simulink model "skarab_adc4x3g_14"  (R2018a)
settings: Solver=VariableStepAuto  StartTime=0.0  StopTime=10.0  RelTol=1e-3
libraries: xbsIndex_r4 x76
settings Model: Creator=qwerty40  LastModifiedBy=clifford
settings CodeAppCC: StateflowObjectComments=on

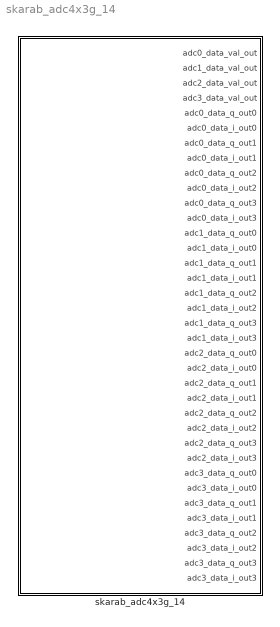
== system skarab_adc4x3g_14 ==
  skarab_adc4x3g_14 : Subsystem  Tag=xps:skarab_adc4x3g_14  mask(hmc){mez=2, sync_ms=Master}
      mask prompts: mez "Mezzanine slot"; sync_ms "Master/Slave"
      mask help: Interface to ADC cards available on SKARAB boards.
      mask init:
      | skarab_adc4x3g_14_mask(gcb);
      mask TypeOptions mez: 0 | 1 | 2 | 3
      mask TypeOptions sync_ms: Master | Slave
      mask DialogControl Container6 Prompt: Parameters

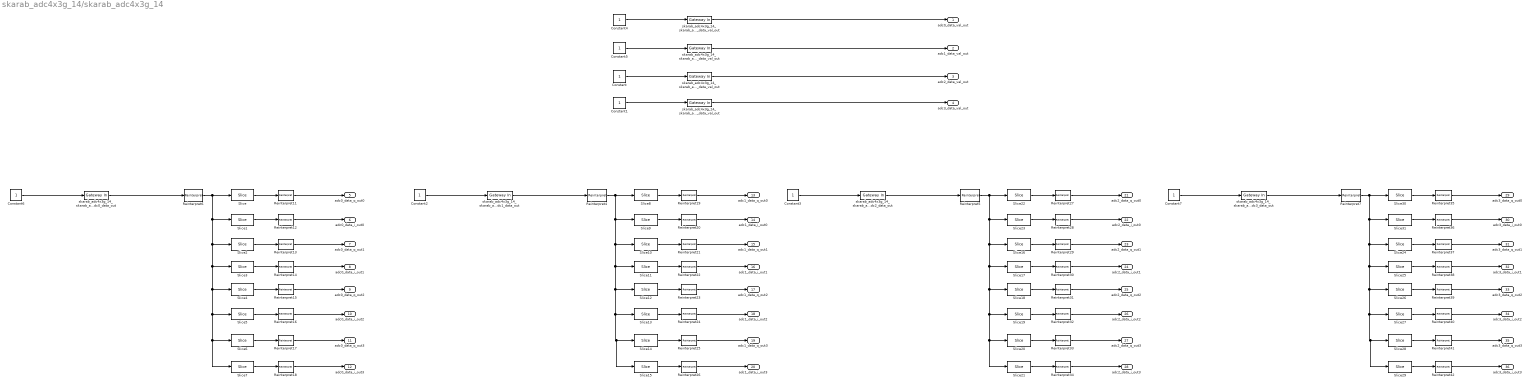
== system skarab_adc4x3g_14/skarab_adc4x3g_14 ==
  Constant{,1..7} (8 alike) : Constant
  Reinterpret{11..42} (32 alike) : xbsIndex_r4/Reinterpret  force_arith_type=on  arith_type="Signed  (2's comp)"  force_bin_pt=on  bin_pt=15  block_type=reinterpret
  Reinterpret{4..7} (4 alike) : xbsIndex_r4/Reinterpret  force_arith_type=on  arith_type=Unsigned  force_bin_pt=on  bin_pt=0  block_type=reinterpret
  Slice{,8,22,30} (4 alike) : xbsIndex_r4/Slice  nbits=16  boolean_output=off  mode=Lower Bit Location + Width  bit1=0  base1=MSB of Input  bit0=0  base0=LSB of Input  dbl_ovrd=off  block_type=slice
  Slice{1,9,23,31} (4 alike) : xbsIndex_r4/Slice  nbits=16  boolean_output=off  mode=Lower Bit Location + Width  bit1=0  base1=MSB of Input  bit0=16  base0=LSB of Input  dbl_ovrd=off  block_type=slice
  Slice{2,10,16,24} (4 alike) : xbsIndex_r4/Slice  nbits=16  boolean_output=off  mode=Lower Bit Location + Width  bit1=0  base1=MSB of Input  bit0=32  base0=LSB of Input  dbl_ovrd=off  block_type=slice
  Slice{3,11,17,25} (4 alike) : xbsIndex_r4/Slice  nbits=16  boolean_output=off  mode=Lower Bit Location + Width  bit1=0  base1=MSB of Input  bit0=48  base0=LSB of Input  dbl_ovrd=off  block_type=slice
  Slice{4,12,18,26} (4 alike) : xbsIndex_r4/Slice  nbits=16  boolean_output=off  mode=Lower Bit Location + Width  bit1=0  base1=MSB of Input  bit0=64  base0=LSB of Input  dbl_ovrd=off  block_type=slice
  Slice{5,13,19,27} (4 alike) : xbsIndex_r4/Slice  nbits=16  boolean_output=off  mode=Lower Bit Location + Width  bit1=0  base1=MSB of Input  bit0=80  base0=LSB of Input  dbl_ovrd=off  block_type=slice
  Slice{6,14,20,28} (4 alike) : xbsIndex_r4/Slice  nbits=16  boolean_output=off  mode=Lower Bit Location + Width  bit1=0  base1=MSB of Input  bit0=96  base0=LSB of Input  dbl_ovrd=off  block_type=slice
  Slice{7,15,21,29} (4 alike) : xbsIndex_r4/Slice  nbits=16  boolean_output=off  mode=Lower Bit Location + Width  bit1=0  base1=MSB of Input  bit0=112  base0=LSB of Input  dbl_ovrd=off  block_type=slice
  skarab_adc4x3g_14_skarab_adc4x3g_14_adc0_data_out : xbsIndex_r4/Gateway In  gui_display_data_type=Fixed-point  arith_type=Unsigned  n_bits=128  bin_pt=0  preci_type=Single  exp_width=8  frac_width=24  rows=1  columns=1  quantization=Truncate  overflow=Wrap  period=1  UseAsADC=off  ADCChannel='1'  interface=None  automatic_assignment=on  address_offset=hex2dec('00')  intf_name=''  intf_description=''  default_value=0  timing_constraint=None  locs_specified=off  LOCs={}  io_standard={}  inherit_from_input=off  hdl_port=on  dbl_ovrd=off  block_type=gatewayin
  skarab_adc4x3g_14_skarab_adc4x3g_14_adc0_data_val_out : xbsIndex_r4/Gateway In  gui_display_data_type=Boolean  arith_type=Boolean  n_bits=16  bin_pt=14  preci_type=Single  exp_width=8  frac_width=24  rows=1  columns=1  quantization="Round  (unbiased: +/- Inf)"  overflow=Saturate  period=1  UseAsADC=off  ADCChannel='1'  interface=None  automatic_assignment=on  address_offset=hex2dec('00')  intf_name=''  intf_description=''  default_value=0  timing_constraint=None  locs_specified=off  LOCs={}  io_standard={}  inherit_from_input=off  hdl_port=on  dbl_ovrd=off  block_type=gatewayin
  skarab_adc4x3g_14_skarab_adc4x3g_14_adc1_data_out : xbsIndex_r4/Gateway In  gui_display_data_type=Fixed-point  arith_type=Unsigned  n_bits=128  bin_pt=0  preci_type=Single  exp_width=8  frac_width=24  rows=1  columns=1  quantization=Truncate  overflow=Wrap  period=1  UseAsADC=off  ADCChannel='1'  interface=None  automatic_assignment=on  address_offset=hex2dec('00')  intf_name=''  intf_description=''  default_value=0  timing_constraint=None  locs_specified=off  LOCs={}  io_standard={}  inherit_from_input=off  hdl_port=on  dbl_ovrd=off  block_type=gatewayin
  skarab_adc4x3g_14_skarab_adc4x3g_14_adc1_data_val_out : xbsIndex_r4/Gateway In  gui_display_data_type=Boolean  arith_type=Boolean  n_bits=16  bin_pt=14  preci_type=Single  exp_width=8  frac_width=24  rows=1  columns=1  quantization="Round  (unbiased: +/- Inf)"  overflow=Saturate  period=1  UseAsADC=off  ADCChannel='1'  interface=None  automatic_assignment=on  address_offset=hex2dec('00')  intf_name=''  intf_description=''  default_value=0  timing_constraint=None  locs_specified=off  LOCs={}  io_standard={}  inherit_from_input=off  hdl_port=on  dbl_ovrd=off  block_type=gatewayin
  skarab_adc4x3g_14_skarab_adc4x3g_14_adc2_data_out : xbsIndex_r4/Gateway In  gui_display_data_type=Fixed-point  arith_type=Unsigned  n_bits=128  bin_pt=0  preci_type=Single  exp_width=8  frac_width=24  rows=1  columns=1  quantization=Truncate  overflow=Wrap  period=1  UseAsADC=off  ADCChannel='1'  interface=None  automatic_assignment=on  address_offset=hex2dec('00')  intf_name=''  intf_description=''  default_value=0  timing_constraint=None  locs_specified=off  LOCs={}  io_standard={}  inherit_from_input=off  hdl_port=on  dbl_ovrd=off  block_type=gatewayin
  skarab_adc4x3g_14_skarab_adc4x3g_14_adc2_data_val_out : xbsIndex_r4/Gateway In  gui_display_data_type=Boolean  arith_type=Boolean  n_bits=16  bin_pt=14  preci_type=Single  exp_width=8  frac_width=24  rows=1  columns=1  quantization="Round  (unbiased: +/- Inf)"  overflow=Saturate  period=1  UseAsADC=off  ADCChannel='1'  interface=None  automatic_assignment=on  address_offset=hex2dec('00')  intf_name=''  intf_description=''  default_value=0  timing_constraint=None  locs_specified=off  LOCs={}  io_standard={}  inherit_from_input=off  hdl_port=on  dbl_ovrd=off  block_type=gatewayin
  skarab_adc4x3g_14_skarab_adc4x3g_14_adc3_data_out : xbsIndex_r4/Gateway In  gui_display_data_type=Fixed-point  arith_type=Unsigned  n_bits=128  bin_pt=0  preci_type=Single  exp_width=8  frac_width=24  rows=1  columns=1  quantization=Truncate  overflow=Wrap  period=1  UseAsADC=off  ADCChannel='1'  interface=None  automatic_assignment=on  address_offset=hex2dec('00')  intf_name=''  intf_description=''  default_value=0  timing_constraint=None  locs_specified=off  LOCs={}  io_standard={}  inherit_from_input=off  hdl_port=on  dbl_ovrd=off  block_type=gatewayin
  skarab_adc4x3g_14_skarab_adc4x3g_14_adc3_data_val_out : xbsIndex_r4/Gateway In  gui_display_data_type=Boolean  arith_type=Boolean  n_bits=16  bin_pt=14  preci_type=Single  exp_width=8  frac_width=24  rows=1  columns=1  quantization="Round  (unbiased: +/- Inf)"  overflow=Saturate  period=1  UseAsADC=off  ADCChannel='1'  interface=None  automatic_assignment=on  address_offset=hex2dec('00')  intf_name=''  intf_description=''  default_value=0  timing_constraint=None  locs_specified=off  LOCs={}  io_standard={}  inherit_from_input=off  hdl_port=on  dbl_ovrd=off  block_type=gatewayin
  adc0_data_val_out : Outport
  adc1_data_val_out : Outport  Port=2
  adc2_data_val_out : Outport  Port=3
  adc3_data_val_out : Outport  Port=4
  adc0_data_q_out0 : Outport  Port=5
  adc0_data_i_out0 : Outport  Port=6
  adc0_data_q_out1 : Outport  Port=7
  adc0_data_i_out1 : Outport  Port=8
  adc0_data_q_out2 : Outport  Port=9
  adc0_data_i_out2 : Outport  Port=10
  adc0_data_q_out3 : Outport  Port=11
  adc0_data_i_out3 : Outport  Port=12
  adc1_data_q_out0 : Outport  Port=13
  adc1_data_i_out0 : Outport  Port=14
  adc1_data_q_out1 : Outport  Port=15
  adc1_data_i_out1 : Outport  Port=16
  adc1_data_q_out2 : Outport  Port=17
  adc1_data_i_out2 : Outport  Port=18
  adc1_data_q_out3 : Outport  Port=19
  adc1_data_i_out3 : Outport  Port=20
  adc2_data_q_out0 : Outport  Port=21
  adc2_data_i_out0 : Outport  Port=22
  adc2_data_q_out1 : Outport  Port=23
  adc2_data_i_out1 : Outport  Port=24
  adc2_data_q_out2 : Outport  Port=25
  adc2_data_i_out2 : Outport  Port=26
  adc2_data_q_out3 : Outport  Port=27
  adc2_data_i_out3 : Outport  Port=28
  adc3_data_q_out0 : Outport  Port=29
  adc3_data_i_out0 : Outport  Port=30
  adc3_data_q_out1 : Outport  Port=31
  adc3_data_i_out1 : Outport  Port=32
  adc3_data_q_out2 : Outport  Port=33
  adc3_data_i_out2 : Outport  Port=34
  adc3_data_q_out3 : Outport  Port=35
  adc3_data_i_out3 : Outport  Port=36
  wires:
  Constant/1 -> skarab_adc4x3g_14_skarab_adc4x3g_14_adc2_data_val_out/1
  skarab_adc4x3g_14_skarab_adc4x3g_14_adc2_data_val_out/1 -> adc2_data_val_out/1
  Constant1/1 -> skarab_adc4x3g_14_skarab_adc4x3g_14_adc3_data_val_out/1
  skarab_adc4x3g_14_skarab_adc4x3g_14_adc3_data_val_out/1 -> adc3_data_val_out/1
  Constant4/1 -> skarab_adc4x3g_14_skarab_adc4x3g_14_adc0_data_val_out/1
  skarab_adc4x3g_14_skarab_adc4x3g_14_adc0_data_val_out/1 -> adc0_data_val_out/1
  Constant5/1 -> skarab_adc4x3g_14_skarab_adc4x3g_14_adc1_data_val_out/1
  skarab_adc4x3g_14_skarab_adc4x3g_14_adc1_data_val_out/1 -> adc1_data_val_out/1
  Constant6/1 -> skarab_adc4x3g_14_skarab_adc4x3g_14_adc0_data_out/1
  skarab_adc4x3g_14_skarab_adc4x3g_14_adc0_data_out/1 -> Reinterpret6/1
  Reinterpret6/1 -> Slice7/1, Slice6/1, Slice5/1, Slice4/1, Slice3/1, Slice2/1, Slice1/1, Slice/1
  Reinterpret11/1 -> adc0_data_q_out0/1
  Slice/1 -> Reinterpret11/1
  Reinterpret12/1 -> adc0_data_i_out0/1
  Slice1/1 -> Reinterpret12/1
  Reinterpret13/1 -> adc0_data_q_out1/1
  Slice2/1 -> Reinterpret13/1
  Reinterpret14/1 -> adc0_data_i_out1/1
  Slice3/1 -> Reinterpret14/1
  Reinterpret15/1 -> adc0_data_q_out2/1
  Slice4/1 -> Reinterpret15/1
  Reinterpret16/1 -> adc0_data_i_out2/1
  Slice5/1 -> Reinterpret16/1
  Reinterpret17/1 -> adc0_data_q_out3/1
  Slice6/1 -> Reinterpret17/1
  Reinterpret18/1 -> adc0_data_i_out3/1
  Slice7/1 -> Reinterpret18/1
  Constant2/1 -> skarab_adc4x3g_14_skarab_adc4x3g_14_adc1_data_out/1
  skarab_adc4x3g_14_skarab_adc4x3g_14_adc1_data_out/1 -> Reinterpret4/1
  Reinterpret4/1 -> Slice15/1, Slice14/1, Slice13/1, Slice12/1, Slice11/1, Slice10/1, Slice9/1, Slice8/1
  Reinterpret19/1 -> adc1_data_q_out0/1
  Slice8/1 -> Reinterpret19/1
  Reinterpret20/1 -> adc1_data_i_out0/1
  Slice9/1 -> Reinterpret20/1
  Reinterpret21/1 -> adc1_data_q_out1/1
  Slice10/1 -> Reinterpret21/1
  Reinterpret22/1 -> adc1_data_i_out1/1
  Slice11/1 -> Reinterpret22/1
  Reinterpret23/1 -> adc1_data_q_out2/1
  Slice12/1 -> Reinterpret23/1
  Reinterpret24/1 -> adc1_data_i_out2/1
  Slice13/1 -> Reinterpret24/1
  Reinterpret25/1 -> adc1_data_q_out3/1
  Slice14/1 -> Reinterpret25/1
  Reinterpret26/1 -> adc1_data_i_out3/1
  Slice15/1 -> Reinterpret26/1
  Constant3/1 -> skarab_adc4x3g_14_skarab_adc4x3g_14_adc2_data_out/1
  skarab_adc4x3g_14_skarab_adc4x3g_14_adc2_data_out/1 -> Reinterpret5/1
  Reinterpret5/1 -> Slice21/1, Slice20/1, Slice19/1, Slice18/1, Slice17/1, Slice16/1, Slice23/1, Slice22/1
  Reinterpret27/1 -> adc2_data_q_out0/1
  Slice22/1 -> Reinterpret27/1
  Reinterpret28/1 -> adc2_data_i_out0/1
  Slice23/1 -> Reinterpret28/1
  Reinterpret29/1 -> adc2_data_q_out1/1
  Slice16/1 -> Reinterpret29/1
  Reinterpret30/1 -> adc2_data_i_out1/1
  Slice17/1 -> Reinterpret30/1
  Reinterpret31/1 -> adc2_data_q_out2/1
  Slice18/1 -> Reinterpret31/1
  Reinterpret32/1 -> adc2_data_i_out2/1
  Slice19/1 -> Reinterpret32/1
  Reinterpret33/1 -> adc2_data_q_out3/1
  Slice20/1 -> Reinterpret33/1
  Reinterpret34/1 -> adc2_data_i_out3/1
  Slice21/1 -> Reinterpret34/1
  Constant7/1 -> skarab_adc4x3g_14_skarab_adc4x3g_14_adc3_data_out/1
  skarab_adc4x3g_14_skarab_adc4x3g_14_adc3_data_out/1 -> Reinterpret7/1
  Reinterpret7/1 -> Slice29/1, Slice28/1, Slice27/1, Slice26/1, Slice25/1, Slice24/1, Slice31/1, Slice30/1
  Reinterpret35/1 -> adc3_data_q_out0/1
  Slice30/1 -> Reinterpret35/1
  Reinterpret36/1 -> adc3_data_i_out0/1
  Slice31/1 -> Reinterpret36/1
  Reinterpret37/1 -> adc3_data_q_out1/1
  Slice24/1 -> Reinterpret37/1
  Reinterpret38/1 -> adc3_data_i_out1/1
  Slice25/1 -> Reinterpret38/1
  Reinterpret39/1 -> adc3_data_q_out2/1
  Slice26/1 -> Reinterpret39/1
  Reinterpret40/1 -> adc3_data_i_out2/1
  Slice27/1 -> Reinterpret40/1
  Reinterpret41/1 -> adc3_data_q_out3/1
  Slice28/1 -> Reinterpret41/1
  Reinterpret42/1 -> adc3_data_i_out3/1
  Slice29/1 -> Reinterpret42/1
